simulink model "discrete_red_dim_observer"  (R2020b)
settings: Solver=VariableStepAuto  StartTime=0.0  StopTime=10.0  RelTol=1e-3
settings Model: Creator=10853  LastModifiedBy=10853

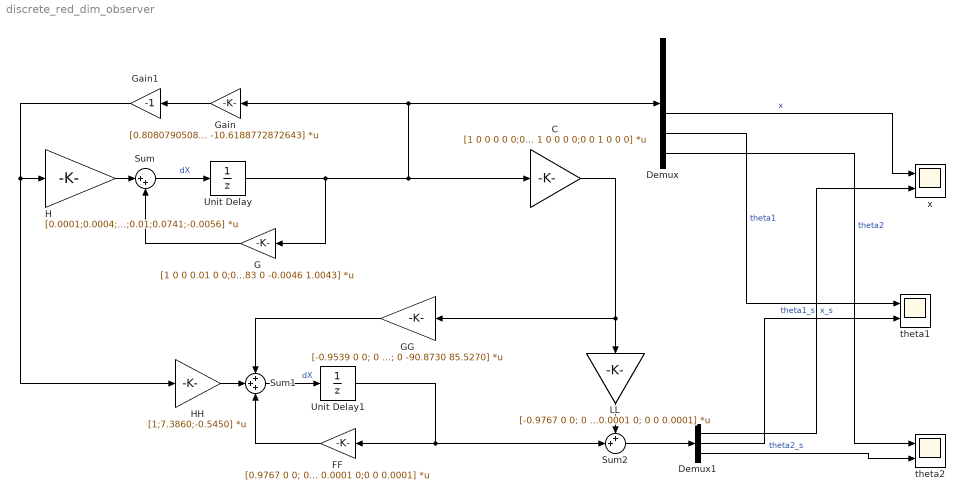
== system discrete_red_dim_observer ==
  C : Gain  Gain=[1 0 0 0 0 0;0 1 0 0 0 0;0 0 1 0 0 0]  Multiplication=Matrix(K*u)
  Demux : Demux  Outputs=6
  Demux1 : Demux  Outputs=3
  FF : Gain  Gain=[0.9767 0 0; 0 0.0001 0;0 0 0.0001]  Multiplication=Matrix(K*u)
  G : Gain  Gain=[1 0 0 0.01 0 0;0 1.0095 -0.0059 0 0.01 0;0 -0.0046 1.0043 0 0 0.01; 0 0 0 1 0 0;0 1.9009 -1.1747 0 1.0095 -0.0059; 0 -0.9129 0.8583 0 -0.0046 1.0043]  Multiplication=Matrix(K*u)
  GG : Gain  Gain=[-0.9539 0 0; 0 189.3180 -116.9320; 0 -90.8730 85.5270]  Multiplication=Matrix(K*u)
  Gain : Gain  Gain=[0.808079050860791 100.847272737157 -106.506186957940 1.59703885887324 4.21261961968780 -10.6188772872643]  Multiplication=Matrix(K*u)
  Gain1 : Gain  Gain=-1
  H : Gain  Gain=[0.0001;0.0004;0;0.01;0.0741;-0.0056]  Multiplication=Matrix(K*u)
  HH : Gain  Gain=[1;7.3860;-0.5450]  Multiplication=Matrix(K*u)
  LL : Gain  Gain=[-0.9767 0 0; 0 0.0001 0; 0 0 0.0001]  Multiplication=Matrix(K*u)
  Sum : Sum  Inputs=|++
  Sum1 : Sum  Inputs=+++
  Sum2 : Sum  Inputs=++|
  Unit Delay : UnitDelay  InitialCondition=[0 pi/36 pi/36 0 0 0]  SampleTime=0.01  HasFrameUpgradeWarning=on
  Unit Delay1 : UnitDelay  InitialCondition=[0 0 0]  SampleTime=0.01  HasFrameUpgradeWarning=on
  theta1 : Scope  NumInputPorts=2
  theta2 : Scope  NumInputPorts=2
  x : Scope  NumInputPorts=2
  wires:
  GG/1 -> Sum1/1
  Demux1/3 -> theta2/2  "theta2_s"
  Gain/1 -> Gain1/1
  Sum1/1 -> Unit Delay1/1  "dX"
  Gain1/1 -> HH/1, H/1
  HH/1 -> Sum1/2
  Unit Delay/1 -> Demux/1, Gain/1, C/1, G/1
  H/1 -> Sum/1
  G/1 -> Sum/2
  Unit Delay1/1 -> Sum2/2, FF/1
  Demux1/2 -> theta1/2  "theta1_s"
  C/1 -> GG/1, LL/1
  Demux1/1 -> x/2  "x_s"
  FF/1 -> Sum1/3
  Sum/1 -> Unit Delay/1  "dX"
  LL/1 -> Sum2/1
  Sum2/1 -> Demux1/1
  Demux/4 -> x/1  "x"
  Demux/5 -> theta1/1  "theta1"
  Demux/6 -> theta2/1  "theta2"
